simulink model "double_step_simFLC"  (R2023b)
settings: Solver=VariableStepAuto  StartTime=0.0  StopTime=18  RelTol=1e-3
libraries: SignalEditorBlockLib x1, fuzblock x1
settings Model: Creator=minakosm  LastModifiedBy=yiannislevy
settings OptimizationCC: ReuseModelBlockBuffer=off

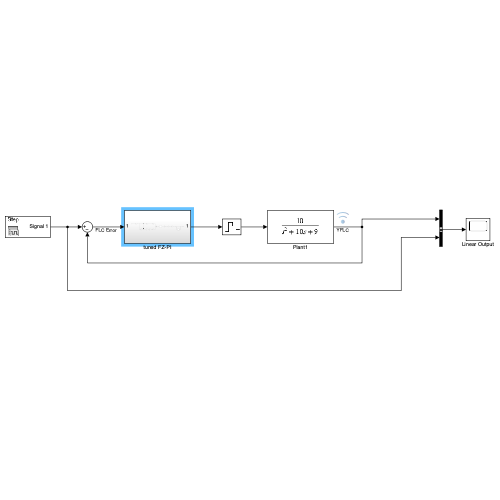
[thumbnail: Simulink's stored preview of the top-level diagram]
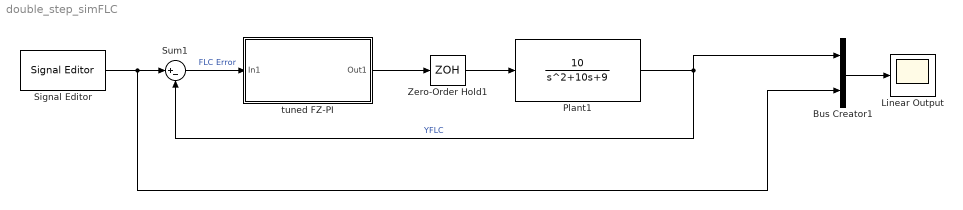
== system double_step_simFLC ==
  Bus Creator1 : BusCreator  Inputs=2
  Linear Output : Scope
  Plant1 : TransferFcn  Numerator=[10]  Denominator=[1 10 9]
  Signal Editor : SignalEditorBlockLib/Signal Editor  FileName=SignalScenarios.mat  ActiveScenario=Step  ActiveSignal=Signal 1  IsBus=off  OutputBusObjectStr=Bus: BusObject  SampleTime=0  ZeroCross=off  OutputAfterFinalValue=Setting to zero  Unit=inherit  PreserveSignalName=on  ApplySigPropsToAllScenarios=on  ApplySigPropsToAllSignals=off
  Sum1 : Sum  Inputs=|+-
  Zero-Order Hold1 : ZeroOrderHold  SampleTime=-1
  tuned FZ-PI : Subsystem
  wires:
  Sum1/1 -> tuned FZ-PI/1(In1)  "FLC Error"
  tuned FZ-PI/1(Out1) -> Zero-Order Hold1/1
  Zero-Order Hold1/1 -> Plant1/1
  Plant1/1 -> Bus Creator1/1, Sum1/2  "YFLC"
  Signal Editor/1 -> Bus Creator1/2, Sum1/1
  Bus Creator1/1 -> Linear Output/1

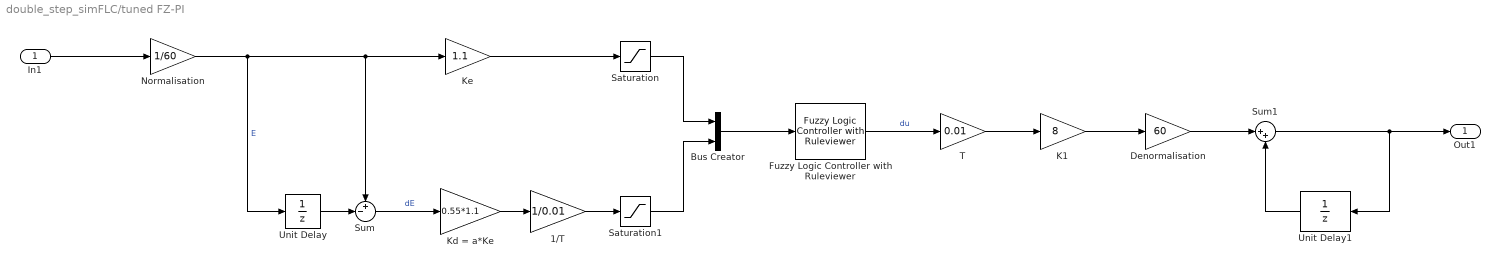
== system double_step_simFLC/tuned FZ-PI ==
  In1 : Inport
  1/T : Gain  Gain=1/0.01
  Bus Creator : BusCreator  Inputs=2
  Denormalisation : Gain  Gain=60
  Fuzzy Logic Controller with Ruleviewer : fuzblock/Fuzzy Logic  Controller  with Ruleviewer  fismatrix=FLC  Ts=0.01
  K1 : Gain  Gain=8
  Kd = a*Ke : Gain  Gain=0.55*1.1
  Ke : Gain  Gain=1.1
  Normalisation : Gain  Gain=1/60
  Saturation : Saturate  UpperLimit=1  LowerLimit=-1
  Saturation1 : Saturate  UpperLimit=1  LowerLimit=-1
  Sum : Sum  Inputs=+-|
  Sum1 : Sum  Inputs=|++
  T : Gain  Gain=0.01
  Unit Delay : UnitDelay  SampleTime=-1  HasFrameUpgradeWarning=on
  Unit Delay1 : UnitDelay  SampleTime=-1  HasFrameUpgradeWarning=on
  Out1 : Outport
  wires:
  In1/1 -> Normalisation/1
  K1/1 -> Denormalisation/1
  Unit Delay/1 -> Sum/2
  Saturation1/1 -> Bus Creator/2
  Sum1/1 -> Out1/1, Unit Delay1/1
  T/1 -> K1/1
  Bus Creator/1 -> Fuzzy Logic Controller with Ruleviewer/1
  1/T/1 -> Saturation1/1
  Fuzzy Logic Controller with Ruleviewer/1 -> T/1  "du"
  Saturation/1 -> Bus Creator/1
  Sum/1 -> Kd = a*Ke/1  "dE"
  Normalisation/1 -> Ke/1, Sum/1, Unit Delay/1  "E"
  Ke/1 -> Saturation/1
  Unit Delay1/1 -> Sum1/2
  Denormalisation/1 -> Sum1/1
  Kd = a*Ke/1 -> 1/T/1
